simulink model "observability"  (R2022b)
settings: Solver=VariableStepAuto  StartTime=0.0  StopTime=10.0  RelTol=1e-3
settings Model: Creator=dmitry  LastModifiedBy=anver
settings OptimizationCC: ReuseModelBlockBuffer=on

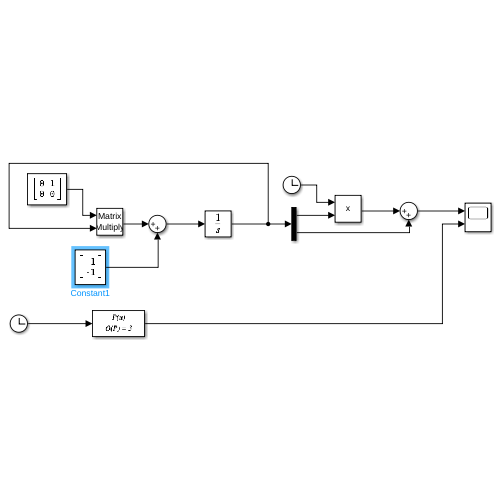
[thumbnail: Simulink's stored preview of the top-level diagram]
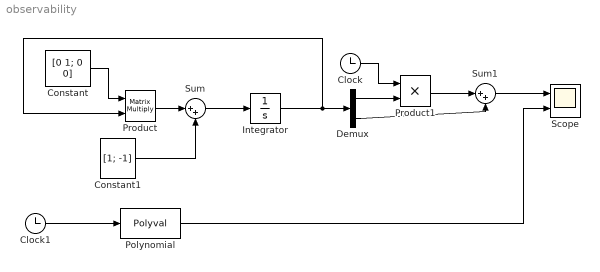
== system observability ==
  Clock : Clock
  Clock1 : Clock
  Constant : Constant  Value=[0 1; 0 0]
  Constant1 : Constant  Value=[1; -1]  VectorParams1D=off
  Demux : Demux  Outputs=2
  Integrator : Integrator
  Polynomial : Polyval  Coefs=[ -1/2, 1. -1. 0]
  Product : Product  Multiplication=Matrix(*)
  Product1 : Product
  Scope : Scope  NumInputPorts=2
  Sum : Sum  Inputs=|++
  Sum1 : Sum  Inputs=|++
  wires:
  Integrator/1 -> Demux/1, Product/2
  Product/1 -> Sum/1
  Constant/1 -> Product/1
  Sum/1 -> Integrator/1
  Constant1/1 -> Sum/2
  Product1/1 -> Sum1/1
  Clock/1 -> Product1/1
  Demux/1 -> Product1/2
  Demux/2 -> Sum1/2
  Sum1/1 -> Scope/1
  Polynomial/1 -> Scope/2
  Clock1/1 -> Polynomial/1
